simulink model "gm_uz_pmsm_model_9ph_working_vnl"  (R2021a)
settings: Solver=FixedStepAuto  StartTime=0.0  StopTime=0.04  RelTol=1e-3
PreLoadFcn:
  | uz_pmsm_model_9ph_init_parameter
undefined symbols (not defined in the file or in its folder): a, b, c, friction_coefficient, inertia, k_i_d, k_p_d, k_p_q, L_d, L_o1, L_o2, L_q, L_x1, L_x2, L_y1, L_y2, L_zero, polepair, psi_pm, R_1, static_friction_torque, ts
libraries: hdlmdlgenlib x182, hdlsllib x92, simulink x15, pid_lib x2
(part 3 of 5)

== system gm_uz_pmsm_model_9ph_working_vnl/Compare/Assert_out_theta_el ==
  cosim : Inport
  dut : Inport  Port=2
  AssertEq : Assertion  StopWhenAssertionFail=off
  Compare To Zero : simulink/Logic and Bit Operations/Compare To Zero  relop===  OutDataTypeStr=boolean
  Constant1 : Constant  Value=0  OutDataTypeStr=Inherit: Inherit via back propagation  SampleTime=-1
  Counter : simulink/Sources/Counter Free-Running  NumBits=32  tsamp=-1
  IgnoreCycles : Constant  Value=2  OutDataTypeStr=Inherit: Inherit via back propagation  SampleTime=-1
  Relational Operator : RelationalOperator  Operator=<  OutDataTypeStr=boolean  RndMeth=Nearest
  Relational Operator1 : RelationalOperator  Operator===  OutDataTypeStr=boolean  RndMeth=Nearest
  Switch : Switch  Criteria=u2 ~= 0
  Switch1 : Switch  Criteria=u2 ~= 0
  compare: out_theta_el : Scope  NumInputPorts=3
  wires:
  Compare To Zero/1 -> compare: out_theta_el/3
  Relational Operator1/1 -> Compare To Zero/1, AssertEq/1  "err"
  Switch1/1 -> compare: out_theta_el/1, Relational Operator1/1
  Switch/1 -> compare: out_theta_el/2, Relational Operator1/2
  Constant1/1 -> Switch/1, Switch1/1
  Relational Operator/1 -> Switch/2, Switch1/2
  cosim/1 -> Switch1/3  "cosim"
  dut/1 -> Switch/3  "dut ref"
  Counter/1 -> Relational Operator/1
  IgnoreCycles/1 -> Relational Operator/2

== system gm_uz_pmsm_model_9ph_working_vnl/Compare/Assert_outputs ==
  cosim : Inport
  dut : Inport  Port=2
  AssertEq : Assertion  StopWhenAssertionFail=off
  Compare To Zero : simulink/Logic and Bit Operations/Compare To Zero  relop===  OutDataTypeStr=boolean
  Constant1 : Constant  Value=0  OutDataTypeStr=Inherit: Inherit via back propagation  SampleTime=-1
  Counter : simulink/Sources/Counter Free-Running  NumBits=32  tsamp=-1
  IgnoreCycles : Constant  Value=2  OutDataTypeStr=Inherit: Inherit via back propagation  SampleTime=-1
  RelErrCheck : Subsystem
  Relational Operator : RelationalOperator  Operator=<  OutDataTypeStr=boolean  RndMeth=Nearest
  Switch : Switch  Criteria=u2 ~= 0
  Switch1 : Switch  Criteria=u2 ~= 0
  compare: outputs : Scope  NumInputPorts=3
  wires:
  IgnoreCycles/1 -> Relational Operator/2
  Counter/1 -> Relational Operator/1
  dut/1 -> Switch/3  "dut ref"
  cosim/1 -> Switch1/3  "cosim"
  Relational Operator/1 -> Switch1/2, Switch/2
  Constant1/1 -> Switch1/1, Switch/1
  Switch/1 -> compare: outputs/2, RelErrCheck/2(In2)
  Switch1/1 -> compare: outputs/1, RelErrCheck/1(In1)
  RelErrCheck/1(Out1) -> AssertEq/1, Compare To Zero/1  "err"
  Compare To Zero/1 -> compare: outputs/3

== system gm_uz_pmsm_model_9ph_working_vnl/Compare/CleanupScopes ==

== system gm_uz_pmsm_model_9ph_working_vnl/Compare/Enable ==

== system gm_uz_pmsm_model_9ph_working_vnl/FOC_controller/decoupling ==
  i_d : Inport
  i_q : Inport  Port=2
  omega_m : Inport  Port=3
  Constant1 : Constant  Value=psi_pm  SampleTime=-1
  Gain : Gain  Gain=L_q
  Gain1 : Gain  Gain=L_d
  Gain2 : Gain  Gain=polepair
  Product : Product
  Product1 : Product
  Sum6 : Sum  Inputs=|++
  u_d : Outport
  u_q : Outport  Port=2
  wires:
  Gain/1 -> Product/1
  Gain2/1 -> Product1/2, Product/2
  Product1/1 -> u_q/1
  i_d/1 -> Gain1/1
  Product/1 -> u_d/1
  Gain1/1 -> Sum6/1
  i_q/1 -> Gain/1
  Constant1/1 -> Sum6/2
  Sum6/1 -> Product1/1
  omega_m/1 -> Gain2/1

== system gm_uz_pmsm_model_9ph_working_vnl/uz_pmsm_model_9ph/Add ==
  In1 : Inport
  In2 : Inport  Port=2
  Add : Sum  Inputs=+-  OutDataTypeStr=single  SampleTime=2e-09
  Add_pd1 : Delay  DelayLength=6
  Out1 : Outport
  wires:
  Add_pd1/1 -> Out1/1
  Add/1 -> Add_pd1/1
  In2/1 -> Add/2
  In1/1 -> Add/1

== system gm_uz_pmsm_model_9ph_working_vnl/uz_pmsm_model_9ph/Add1 ==
  In1 : Inport
  In2 : Inport  Port=2
  Add1 : Sum  Inputs=+-  OutDataTypeStr=single  SampleTime=2e-09
  Add1_pd1 : Delay  DelayLength=6
  Out1 : Outport
  wires:
  Add1_pd1/1 -> Out1/1
  Add1/1 -> Add1_pd1/1
  In2/1 -> Add1/2
  In1/1 -> Add1/1

== system gm_uz_pmsm_model_9ph_working_vnl/uz_pmsm_model_9ph/Add2 ==
  In1 : Inport
  In2 : Inport  Port=2
  Add2 : Sum  Inputs=+-  OutDataTypeStr=single  SampleTime=2e-09
  Add2_pd1 : Delay  DelayLength=6
  Out1 : Outport
  wires:
  Add2_pd1/1 -> Out1/1
  Add2/1 -> Add2_pd1/1
  In2/1 -> Add2/2
  In1/1 -> Add2/1

== system gm_uz_pmsm_model_9ph_working_vnl/uz_pmsm_model_9ph/Add3 ==
  In1 : Inport
  In2 : Inport  Port=2
  Add3 : Sum  Inputs=+-  OutDataTypeStr=single  SampleTime=2e-09
  Add3_pd1 : Delay  DelayLength=6
  Out1 : Outport
  wires:
  Add3_pd1/1 -> Out1/1
  Add3/1 -> Add3_pd1/1
  In2/1 -> Add3/2
  In1/1 -> Add3/1

== system gm_uz_pmsm_model_9ph_working_vnl/uz_pmsm_model_9ph/Add4 ==
  In1 : Inport
  In2 : Inport  Port=2
  Add4 : Sum  Inputs=+-  OutDataTypeStr=single  SampleTime=2e-09
  Add4_pd1 : Delay  DelayLength=6
  Out1 : Outport
  wires:
  Add4_pd1/1 -> Out1/1
  Add4/1 -> Add4_pd1/1
  In2/1 -> Add4/2
  In1/1 -> Add4/1

== system gm_uz_pmsm_model_9ph_working_vnl/uz_pmsm_model_9ph/Add5 ==
  In1 : Inport
  In2 : Inport  Port=2
  Add5 : Sum  Inputs=+-  OutDataTypeStr=single  SampleTime=2e-09
  Add5_pd1 : Delay  DelayLength=6
  Out1 : Outport
  wires:
  Add5_pd1/1 -> Out1/1
  Add5/1 -> Add5_pd1/1
  In2/1 -> Add5/2
  In1/1 -> Add5/1

== system gm_uz_pmsm_model_9ph_working_vnl/uz_pmsm_model_9ph/Add6 ==
  In1 : Inport
  In2 : Inport  Port=2
  Add6 : Sum  Inputs=+-  OutDataTypeStr=single  SampleTime=2e-09
  Add6_pd1 : Delay  DelayLength=6
  Out1 : Outport
  wires:
  Add6_pd1/1 -> Out1/1
  Add6/1 -> Add6_pd1/1
  In2/1 -> Add6/2
  In1/1 -> Add6/1

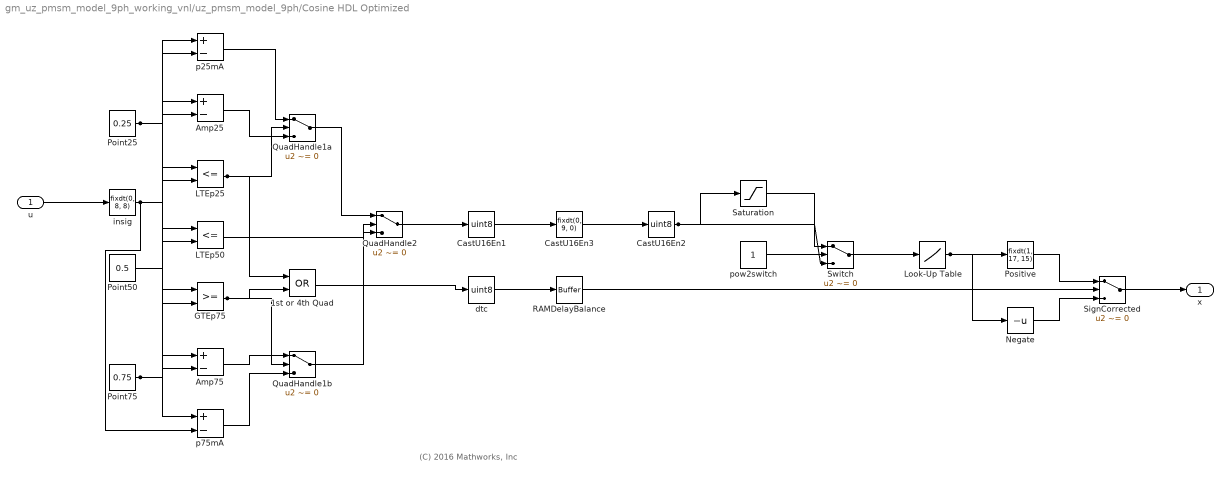
== system gm_uz_pmsm_model_9ph_working_vnl/uz_pmsm_model_9ph/Cosine HDL Optimized ==
  note: (C) 2016 Mathworks, Inc
  u : Inport  OutDataTypeStr=fixdt(1, 25, 12)  SampleTime=2e-09
  1st or 4th Quad : Logic  Operator=OR  AllPortsSameDT=off  OutDataTypeStr=boolean  SampleTime=2e-09
  Amp25 : Sum  Inputs=+-  AccumDataTypeStr=fixdt(1, 18, 17)  OutDataTypeStr=fixdt(1, 18, 17)  SampleTime=2e-09
  Amp75 : Sum  Inputs=+-  AccumDataTypeStr=fixdt(1, 18, 17)  OutDataTypeStr=fixdt(1, 18, 17)  SampleTime=2e-09
  CastU16En1 : DataTypeConversion  OutDataTypeStr=uint8  ConvertRealWorld=Stored Integer (SI)  SampleTime=2e-09
  CastU16En2 : DataTypeConversion  OutDataTypeStr=uint8  ConvertRealWorld=Stored Integer (SI)  SampleTime=2e-09  SaturateOnIntegerOverflow=on
  CastU16En3 : DataTypeConversion  OutDataTypeStr=fixdt(0, 9, 0)  SampleTime=2e-09
  GTEp75 : RelationalOperator  OutDataTypeStr=boolean  SampleTime=2e-09  RndMeth=Nearest
  LTEp25 : RelationalOperator  Operator=<=  OutDataTypeStr=boolean  SampleTime=2e-09  RndMeth=Nearest
  LTEp50 : RelationalOperator  Operator=<=  OutDataTypeStr=boolean  SampleTime=2e-09  RndMeth=Nearest
  Look-Up Table : Lookup_n-D  NumberOfTableDimensions=1  BreakpointsForDimension1="fi(\"numerictype\",numerictype(0,8,0),\"fimath\",fimath(\"RoundingMethod\", \"Floor\",\"OverflowAction\", \"Wrap\",\"ProductMode\",\"FullPrecision\",\"SumMode\",\"FullPrecision\"),\"Value\",\"[0 1 2 3 4 5 6 7 8 9 10 11 12 13 14 15 16 17 18 19 20 21 22 23 24 25 26 27 28 29 30 31 32 33 34 35 36 37 38 39 40 41 42 43 44 45 46 47 48 49 50 51 52 53 54 55 56 57 58 59 60 61 62 63]\")"  Table="reshape(fi(\"numerictype\",numerictype(1,17,15),\"fimath\",fimath(\"RoundingMethod\", \"Floor\",\"OverflowAction\", \"Wrap\",\"ProductMode\",\"FullPrecision\",\"SumMode\",\"FullPrecision\"),\"Value\",\"[0;0.0245361328125;0.049072265625;0.073577880859375;0.0980224609375;0.122406005859375;0.146728515625;0.17095947265625;0.195098876953125;0.2191162109375;0.24298095703125;0.2667236328125;0.290283203125;0.313690185546875;0.336883544921875;0.359893798828125;0.3826904296875;0.405242919921875;0.42755126953125;0.449615478515625;0.471405029296875;0.492889404296875;0.51409912109375;0.535003662109375;0.555572509765625;0.5758056640625;0.595703125;0.615234375;0.6343994140625;0.653167724609375;0.67156982421875;0.689544677734375;0.70709228515625;0.7242431640625;0.740936279296875;0.7572021484375;0.77301025390625;0.788360595703125;0.80322265625;0.817596435546875;0.83148193359375;0.8448486328125;0.85772705078125;0.870086669921875;0.881927490234375;0.893218994140625;0.90399169921875;0.914215087890625;0.92388916015625;0.9329833984375;0.941558837890625;0.94952392578125;0.956939697265625;0.963775634765625;0.97003173828125;0.9757080078125;0.98077392578125;0.98529052734375;0.989166259765625;0.99249267578125;0.99517822265625;0.997283935546875;0.998809814453125;0.99969482421875]\"), [1  64])"  InterpMethod=Flat  ExtrapMethod=Clip  DiagnosticForOutOfRangeInput=Error  SampleTime=2e-09  OutDataTypeStr=fixdt(1, 17, 15)  InputSameDT=on
  Negate : UnaryMinus  SampleTime=2e-09
  Point25 : Constant  Value=0.25  OutDataTypeStr=fixdt(0, 17, 17)  SampleTime=2e-09
  Point50 : Constant  Value=0.5  OutDataTypeStr=fixdt(0, 17, 17)  SampleTime=2e-09
  Point75 : Constant  Value=0.75  OutDataTypeStr=fixdt(0, 17, 17)  SampleTime=2e-09
  Positive : DataTypeConversion  OutDataTypeStr=fixdt(1, 17, 15)  SampleTime=2e-09
  QuadHandle1a : Switch  Criteria=u2 ~= 0  Threshold=double(0)  OutDataTypeStr=fixdt(1, 18, 17)  SampleTime=2e-09
  QuadHandle1b : Switch  Criteria=u2 ~= 0  Threshold=double(0)  OutDataTypeStr=fixdt(1, 18, 17)  SampleTime=2e-09
  QuadHandle2 : Switch  Criteria=u2 ~= 0  Threshold=double(0)  OutDataTypeStr=fixdt(0, 8, 8)  SampleTime=2e-09  SaturateOnIntegerOverflow=on
  RAMDelayBalance : hdlmdlgenlib/Buffer
      settings: SourceProductBaseCode=SL
  Saturation : Saturate  UpperLimit="fi(0,0,8,0,\"hex\",\"3f\")"  LowerLimit="fi(0,0,8,0,\"hex\",\"00\")"  SampleTime=2e-09  OutDataTypeStr=uint8
  SignCorrected : Switch  Criteria=u2 ~= 0  Threshold=double(0)  OutDataTypeStr=fixdt(1, 17, 15)  SampleTime=2e-09
  Switch : Switch  Criteria=u2 ~= 0  Threshold=double(0)  OutDataTypeStr=uint8  SampleTime=2e-09
  dtc : DataTypeConversion  OutDataTypeStr=uint8  SampleTime=2e-09
  insig : DataTypeConversion  OutDataTypeStr=fixdt(0, 8, 8)  SampleTime=2e-09
  p25mA : Sum  Inputs=+-  AccumDataTypeStr=fixdt(1, 18, 17)  OutDataTypeStr=fixdt(1, 18, 17)  SampleTime=2e-09
  p75mA : Sum  Inputs=+-  AccumDataTypeStr=fixdt(1, 18, 17)  OutDataTypeStr=fixdt(1, 18, 17)  SampleTime=2e-09
  pow2switch : Constant  OutDataTypeStr=boolean  SampleTime=2e-09
  x : Outport  SampleTime=2e-09
  wires:
  u/1 -> insig/1
  1st or 4th Quad/1 -> dtc/1
  pow2switch/1 -> Switch/2
  p75mA/1 -> QuadHandle1b/3
  p25mA/1 -> QuadHandle1a/1
  insig/1 -> Amp25/1, Amp75/1, GTEp75/1, LTEp25/1, LTEp50/1, p25mA/2, p75mA/2
  Switch/1 -> Look-Up Table/1
  SignCorrected/1 -> x/1
  Saturation/1 -> Switch/1
  RAMDelayBalance/1 -> SignCorrected/2
  QuadHandle2/1 -> CastU16En1/1
  QuadHandle1b/1 -> QuadHandle2/3
  QuadHandle1a/1 -> QuadHandle2/1
  Positive/1 -> SignCorrected/1
  Point75/1 -> Amp75/2, GTEp75/2, p75mA/1
  Point50/1 -> LTEp50/2
  Point25/1 -> Amp25/2, LTEp25/2, p25mA/1
  Negate/1 -> SignCorrected/3
  Look-Up Table/1 -> Negate/1, Positive/1
  LTEp50/1 -> QuadHandle2/2
  LTEp25/1 -> 1st or 4th Quad/1, QuadHandle1a/2
  GTEp75/1 -> 1st or 4th Quad/2, QuadHandle1b/2
  CastU16En3/1 -> CastU16En2/1
  CastU16En2/1 -> Saturation/1, Switch/3
  CastU16En1/1 -> CastU16En3/1
  Amp75/1 -> QuadHandle1b/1
  Amp25/1 -> QuadHandle1a/3
  dtc/1 -> RAMDelayBalance/1

== system gm_uz_pmsm_model_9ph_working_vnl/uz_pmsm_model_9ph/Data Type Conversion1 ==
  In1 : Inport
  Data Type Conversion1 : DataTypeConversion  OutDataTypeStr=fixdt(1, 25, 12)  RndMeth=Nearest  SampleTime=2e-09
  Data Type Conversion1_pd1 : Delay  DelayLength=6
  Out1 : Outport
  wires:
  Data Type Conversion1_pd1/1 -> Out1/1
  Data Type Conversion1/1 -> Data Type Conversion1_pd1/1
  In1/1 -> Data Type Conversion1/1

== system gm_uz_pmsm_model_9ph_working_vnl/uz_pmsm_model_9ph/Data Type Conversion11 ==
  In1 : Inport
  Data Type Conversion11 : DataTypeConversion  OutDataTypeStr=double  RndMeth=Nearest  SampleTime=2e-09
  Data Type Conversion11_pd1 : Delay  DelayLength=3
  Out1 : Outport
  wires:
  Data Type Conversion11_pd1/1 -> Out1/1
  Data Type Conversion11/1 -> Data Type Conversion11_pd1/1
  In1/1 -> Data Type Conversion11/1

== system gm_uz_pmsm_model_9ph_working_vnl/uz_pmsm_model_9ph/Data Type Conversion13 ==
  In1 : Inport
  Data Type Conversion13 : DataTypeConversion  OutDataTypeStr=single  RndMeth=Nearest  SampleTime=2e-09
  Data Type Conversion13_pd1 : Delay  DelayLength=3
  Out1 : Outport
  wires:
  Data Type Conversion13_pd1/1 -> Out1/1
  Data Type Conversion13/1 -> Data Type Conversion13_pd1/1
  In1/1 -> Data Type Conversion13/1

== system gm_uz_pmsm_model_9ph_working_vnl/uz_pmsm_model_9ph/Data Type Conversion14 ==
  In1 : Inport
  Data Type Conversion14 : DataTypeConversion  OutDataTypeStr=single  RndMeth=Nearest  SampleTime=2e-09
  Data Type Conversion14_pd1 : Delay  DelayLength=3
  Out1 : Outport
  wires:
  Data Type Conversion14_pd1/1 -> Out1/1
  Data Type Conversion14/1 -> Data Type Conversion14_pd1/1
  In1/1 -> Data Type Conversion14/1

== system gm_uz_pmsm_model_9ph_working_vnl/uz_pmsm_model_9ph/Data Type Conversion15 ==
  In1 : Inport
  Data Type Conversion15 : DataTypeConversion  OutDataTypeStr=single  RndMeth=Nearest  SampleTime=2e-09
  Data Type Conversion15_pd1 : Delay  DelayLength=3
  Out1 : Outport
  wires:
  Data Type Conversion15_pd1/1 -> Out1/1
  Data Type Conversion15/1 -> Data Type Conversion15_pd1/1
  In1/1 -> Data Type Conversion15/1

== system gm_uz_pmsm_model_9ph_working_vnl/uz_pmsm_model_9ph/Data Type Conversion16 ==
  In1 : Inport
  Data Type Conversion16 : DataTypeConversion  OutDataTypeStr=single  RndMeth=Nearest  SampleTime=2e-09
  Data Type Conversion16_pd1 : Delay  DelayLength=3
  Out1 : Outport
  wires:
  Data Type Conversion16_pd1/1 -> Out1/1
  Data Type Conversion16/1 -> Data Type Conversion16_pd1/1
  In1/1 -> Data Type Conversion16/1

== system gm_uz_pmsm_model_9ph_working_vnl/uz_pmsm_model_9ph/Data Type Conversion17 ==
  In1 : Inport
  Data Type Conversion17 : DataTypeConversion  OutDataTypeStr=single  RndMeth=Nearest  SampleTime=2e-09
  Data Type Conversion17_pd1 : Delay  DelayLength=3
  Out1 : Outport
  wires:
  Data Type Conversion17_pd1/1 -> Out1/1
  Data Type Conversion17/1 -> Data Type Conversion17_pd1/1
  In1/1 -> Data Type Conversion17/1

== system gm_uz_pmsm_model_9ph_working_vnl/uz_pmsm_model_9ph/Data Type Conversion18 ==
  In1 : Inport
  Data Type Conversion18 : DataTypeConversion  OutDataTypeStr=single  RndMeth=Nearest  SampleTime=2e-09
  Data Type Conversion18_pd1 : Delay  DelayLength=3
  Out1 : Outport
  wires:
  Data Type Conversion18_pd1/1 -> Out1/1
  Data Type Conversion18/1 -> Data Type Conversion18_pd1/1
  In1/1 -> Data Type Conversion18/1

== system gm_uz_pmsm_model_9ph_working_vnl/uz_pmsm_model_9ph/Data Type Conversion19 ==
  In1 : Inport
  Data Type Conversion19 : DataTypeConversion  OutDataTypeStr=single  RndMeth=Nearest  SampleTime=2e-09
  Data Type Conversion19_pd1 : Delay  DelayLength=3
  Out1 : Outport
  wires:
  Data Type Conversion19_pd1/1 -> Out1/1
  Data Type Conversion19/1 -> Data Type Conversion19_pd1/1
  In1/1 -> Data Type Conversion19/1

== system gm_uz_pmsm_model_9ph_working_vnl/uz_pmsm_model_9ph/Data Type Conversion20 ==
  In1 : Inport
  Data Type Conversion20 : DataTypeConversion  OutDataTypeStr=single  RndMeth=Nearest  SampleTime=2e-09
  Data Type Conversion20_pd1 : Delay  DelayLength=3
  Out1 : Outport
  wires:
  Data Type Conversion20_pd1/1 -> Out1/1
  Data Type Conversion20/1 -> Data Type Conversion20_pd1/1
  In1/1 -> Data Type Conversion20/1

== system gm_uz_pmsm_model_9ph_working_vnl/uz_pmsm_model_9ph/Data Type Conversion21 ==
  In1 : Inport
  Data Type Conversion21 : DataTypeConversion  OutDataTypeStr=double  RndMeth=Nearest  SampleTime=2e-09
  Data Type Conversion21_pd1 : Delay  DelayLength=3
  Out1 : Outport
  wires:
  Data Type Conversion21_pd1/1 -> Out1/1
  Data Type Conversion21/1 -> Data Type Conversion21_pd1/1
  In1/1 -> Data Type Conversion21/1

== system gm_uz_pmsm_model_9ph_working_vnl/uz_pmsm_model_9ph/Data Type Conversion22 ==
  In1 : Inport
  Data Type Conversion22 : DataTypeConversion  OutDataTypeStr=single  RndMeth=Nearest  SampleTime=2e-09
  Data Type Conversion22_pd1 : Delay  DelayLength=6
  Out1 : Outport
  wires:
  Data Type Conversion22_pd1/1 -> Out1/1
  Data Type Conversion22/1 -> Data Type Conversion22_pd1/1
  In1/1 -> Data Type Conversion22/1

== system gm_uz_pmsm_model_9ph_working_vnl/uz_pmsm_model_9ph/Data Type Conversion221 ==
  In1 : Inport
  Data Type Conversion221 : DataTypeConversion  OutDataTypeStr=double  RndMeth=Nearest  SampleTime=2e-09
  Data Type Conversion221_pd1 : Delay  DelayLength=3
  Out1 : Outport
  wires:
  Data Type Conversion221_pd1/1 -> Out1/1
  Data Type Conversion221/1 -> Data Type Conversion221_pd1/1
  In1/1 -> Data Type Conversion221/1

== system gm_uz_pmsm_model_9ph_working_vnl/uz_pmsm_model_9ph/Data Type Conversion23 ==
  In1 : Inport
  Data Type Conversion23 : DataTypeConversion  OutDataTypeStr=single  RndMeth=Nearest  SampleTime=2e-09
  Data Type Conversion23_pd1 : Delay  DelayLength=3
  Out1 : Outport
  wires:
  Data Type Conversion23_pd1/1 -> Out1/1
  Data Type Conversion23/1 -> Data Type Conversion23_pd1/1
  In1/1 -> Data Type Conversion23/1

== system gm_uz_pmsm_model_9ph_working_vnl/uz_pmsm_model_9ph/Data Type Conversion24 ==
  In1 : Inport
  Data Type Conversion24 : DataTypeConversion  OutDataTypeStr=double  RndMeth=Nearest  SampleTime=2e-09
  Data Type Conversion24_pd1 : Delay  DelayLength=3
  Out1 : Outport
  wires:
  Data Type Conversion24_pd1/1 -> Out1/1
  Data Type Conversion24/1 -> Data Type Conversion24_pd1/1
  In1/1 -> Data Type Conversion24/1

== system gm_uz_pmsm_model_9ph_working_vnl/uz_pmsm_model_9ph/Data Type Conversion25 ==
  In1 : Inport
  Data Type Conversion25 : DataTypeConversion  OutDataTypeStr=double  RndMeth=Nearest  SampleTime=2e-09
  Data Type Conversion25_pd1 : Delay  DelayLength=3
  Out1 : Outport
  wires:
  Data Type Conversion25_pd1/1 -> Out1/1
  Data Type Conversion25/1 -> Data Type Conversion25_pd1/1
  In1/1 -> Data Type Conversion25/1

== system gm_uz_pmsm_model_9ph_working_vnl/uz_pmsm_model_9ph/Data Type Conversion26 ==
  In1 : Inport
  Data Type Conversion26 : DataTypeConversion  OutDataTypeStr=double  RndMeth=Nearest  SampleTime=2e-09
  Data Type Conversion26_pd1 : Delay  DelayLength=3
  Out1 : Outport
  wires:
  Data Type Conversion26_pd1/1 -> Out1/1
  Data Type Conversion26/1 -> Data Type Conversion26_pd1/1
  In1/1 -> Data Type Conversion26/1

== system gm_uz_pmsm_model_9ph_working_vnl/uz_pmsm_model_9ph/Data Type Conversion27 ==
  In1 : Inport
  Data Type Conversion27 : DataTypeConversion  OutDataTypeStr=double  RndMeth=Nearest  SampleTime=2e-09
  Data Type Conversion27_pd1 : Delay  DelayLength=3
  Out1 : Outport
  wires:
  Data Type Conversion27_pd1/1 -> Out1/1
  Data Type Conversion27/1 -> Data Type Conversion27_pd1/1
  In1/1 -> Data Type Conversion27/1

== system gm_uz_pmsm_model_9ph_working_vnl/uz_pmsm_model_9ph/Data Type Conversion28 ==
  In1 : Inport
  Data Type Conversion28 : DataTypeConversion  OutDataTypeStr=double  RndMeth=Nearest  SampleTime=2e-09
  Data Type Conversion28_pd1 : Delay  DelayLength=3
  Out1 : Outport
  wires:
  Data Type Conversion28_pd1/1 -> Out1/1
  Data Type Conversion28/1 -> Data Type Conversion28_pd1/1
  In1/1 -> Data Type Conversion28/1

== system gm_uz_pmsm_model_9ph_working_vnl/uz_pmsm_model_9ph/Data Type Conversion29 ==
  In1 : Inport
  Data Type Conversion29 : DataTypeConversion  OutDataTypeStr=double  RndMeth=Nearest  SampleTime=2e-09
  Data Type Conversion29_pd1 : Delay  DelayLength=3
  Out1 : Outport
  wires:
  Data Type Conversion29_pd1/1 -> Out1/1
  Data Type Conversion29/1 -> Data Type Conversion29_pd1/1
  In1/1 -> Data Type Conversion29/1

== system gm_uz_pmsm_model_9ph_working_vnl/uz_pmsm_model_9ph/Data Type Conversion30 ==
  In1 : Inport
  Data Type Conversion30 : DataTypeConversion  OutDataTypeStr=double  RndMeth=Nearest  SampleTime=2e-09
  Data Type Conversion30_pd1 : Delay  DelayLength=3
  Out1 : Outport
  wires:
  Data Type Conversion30_pd1/1 -> Out1/1
  Data Type Conversion30/1 -> Data Type Conversion30_pd1/1
  In1/1 -> Data Type Conversion30/1

== system gm_uz_pmsm_model_9ph_working_vnl/uz_pmsm_model_9ph/Data Type Conversion32 ==
  In1 : Inport
  Data Type Conversion32 : DataTypeConversion  OutDataTypeStr=single  RndMeth=Nearest  SampleTime=2e-09
  Data Type Conversion32_pd1 : Delay  DelayLength=6
  Out1 : Outport
  wires:
  Data Type Conversion32_pd1/1 -> Out1/1
  Data Type Conversion32/1 -> Data Type Conversion32_pd1/1
  In1/1 -> Data Type Conversion32/1

== system gm_uz_pmsm_model_9ph_working_vnl/uz_pmsm_model_9ph/Data Type Conversion8 ==
  In1 : Inport
  Data Type Conversion8 : DataTypeConversion  OutDataTypeStr=single  RndMeth=Nearest  SampleTime=2e-09
  Data Type Conversion8_pd1 : Delay  DelayLength=3
  Out1 : Outport
  wires:
  Data Type Conversion8_pd1/1 -> Out1/1
  Data Type Conversion8/1 -> Data Type Conversion8_pd1/1
  In1/1 -> Data Type Conversion8/1

== system gm_uz_pmsm_model_9ph_working_vnl/uz_pmsm_model_9ph/Divide ==
  In1 : Inport
  In2 : Inport  Port=2
  Divide : Product  Inputs=**  OutDataTypeStr=single  SampleTime=2e-09
  Divide_pd1 : Delay  DelayLength=6
  Out1 : Outport
  wires:
  Divide_pd1/1 -> Out1/1
  Divide/1 -> Divide_pd1/1
  In2/1 -> Divide/2
  In1/1 -> Divide/1

== system gm_uz_pmsm_model_9ph_working_vnl/uz_pmsm_model_9ph/Divide1 ==
  In1 : Inport
  In2 : Inport  Port=2
  Divide1 : Product  Inputs=**  OutDataTypeStr=single  SampleTime=2e-09
  Divide1_pd1 : Delay  DelayLength=6
  Out1 : Outport
  wires:
  Divide1_pd1/1 -> Out1/1
  Divide1/1 -> Divide1_pd1/1
  In2/1 -> Divide1/2
  In1/1 -> Divide1/1

== system gm_uz_pmsm_model_9ph_working_vnl/uz_pmsm_model_9ph/Divide10 ==
  In1 : Inport
  In2 : Inport  Port=2
  Divide10 : Product  Inputs=**  OutDataTypeStr=single  SampleTime=2e-09
  Divide10_pd1 : Delay  DelayLength=6
  Out1 : Outport
  wires:
  Divide10_pd1/1 -> Out1/1
  Divide10/1 -> Divide10_pd1/1
  In2/1 -> Divide10/2
  In1/1 -> Divide10/1

== system gm_uz_pmsm_model_9ph_working_vnl/uz_pmsm_model_9ph/Divide11 ==
  In1 : Inport
  In2 : Inport  Port=2
  Divide11 : Product  Inputs=**  OutDataTypeStr=single  SampleTime=2e-09
  Divide11_pd1 : Delay  DelayLength=6
  Out1 : Outport
  wires:
  Divide11_pd1/1 -> Out1/1
  Divide11/1 -> Divide11_pd1/1
  In2/1 -> Divide11/2
  In1/1 -> Divide11/1

== system gm_uz_pmsm_model_9ph_working_vnl/uz_pmsm_model_9ph/Divide12 ==
  In1 : Inport
  In2 : Inport  Port=2
  Divide12 : Product  Inputs=**  OutDataTypeStr=single  SampleTime=2e-09
  Divide12_pd1 : Delay  DelayLength=6
  Out1 : Outport
  wires:
  Divide12_pd1/1 -> Out1/1
  Divide12/1 -> Divide12_pd1/1
  In2/1 -> Divide12/2
  In1/1 -> Divide12/1

== system gm_uz_pmsm_model_9ph_working_vnl/uz_pmsm_model_9ph/Divide13 ==
  In1 : Inport
  In2 : Inport  Port=2
  Divide13 : Product  Inputs=**  OutDataTypeStr=single  SampleTime=2e-09
  Divide13_pd1 : Delay  DelayLength=6
  Out1 : Outport
  wires:
  Divide13_pd1/1 -> Out1/1
  Divide13/1 -> Divide13_pd1/1
  In2/1 -> Divide13/2
  In1/1 -> Divide13/1

== system gm_uz_pmsm_model_9ph_working_vnl/uz_pmsm_model_9ph/Divide2 ==
  In1 : Inport
  In2 : Inport  Port=2
  Divide2 : Product  Inputs=**  OutDataTypeStr=single  SampleTime=2e-09
  Divide2_pd1 : Delay  DelayLength=6
  Out1 : Outport
  wires:
  Divide2_pd1/1 -> Out1/1
  Divide2/1 -> Divide2_pd1/1
  In2/1 -> Divide2/2
  In1/1 -> Divide2/1

== system gm_uz_pmsm_model_9ph_working_vnl/uz_pmsm_model_9ph/Divide3 ==
  In1 : Inport
  In2 : Inport  Port=2
  Divide3 : Product  Inputs=**  OutDataTypeStr=single  SampleTime=2e-09
  Divide3_pd1 : Delay  DelayLength=6
  Out1 : Outport
  wires:
  Divide3_pd1/1 -> Out1/1
  Divide3/1 -> Divide3_pd1/1
  In2/1 -> Divide3/2
  In1/1 -> Divide3/1

== system gm_uz_pmsm_model_9ph_working_vnl/uz_pmsm_model_9ph/Divide4 ==
  In1 : Inport
  In2 : Inport  Port=2
  Divide4 : Product  Inputs=**  OutDataTypeStr=single  SampleTime=2e-09
  Divide4_pd1 : Delay  DelayLength=6
  Out1 : Outport
  wires:
  Divide4_pd1/1 -> Out1/1
  Divide4/1 -> Divide4_pd1/1
  In2/1 -> Divide4/2
  In1/1 -> Divide4/1

== system gm_uz_pmsm_model_9ph_working_vnl/uz_pmsm_model_9ph/Divide5 ==
  In1 : Inport
  In2 : Inport  Port=2
  Divide5 : Product  Inputs=**  OutDataTypeStr=single  SampleTime=2e-09
  Divide5_pd1 : Delay  DelayLength=6
  Out1 : Outport
  wires:
  Divide5_pd1/1 -> Out1/1
  Divide5/1 -> Divide5_pd1/1
  In2/1 -> Divide5/2
  In1/1 -> Divide5/1

== system gm_uz_pmsm_model_9ph_working_vnl/uz_pmsm_model_9ph/Divide6 ==
  In1 : Inport
  In2 : Inport  Port=2
  Divide6 : Product  Inputs=**  OutDataTypeStr=single  SampleTime=2e-09
  Divide6_pd1 : Delay  DelayLength=6
  Out1 : Outport
  wires:
  Divide6_pd1/1 -> Out1/1
  Divide6/1 -> Divide6_pd1/1
  In2/1 -> Divide6/2
  In1/1 -> Divide6/1

== system gm_uz_pmsm_model_9ph_working_vnl/uz_pmsm_model_9ph/Divide7 ==
  In1 : Inport
  In2 : Inport  Port=2
  Divide7 : Product  Inputs=**  OutDataTypeStr=single  SampleTime=2e-09
  Divide7_pd1 : Delay  DelayLength=6
  Out1 : Outport
  wires:
  Divide7_pd1/1 -> Out1/1
  Divide7/1 -> Divide7_pd1/1
  In2/1 -> Divide7/2
  In1/1 -> Divide7/1

== system gm_uz_pmsm_model_9ph_working_vnl/uz_pmsm_model_9ph/Divide8 ==
  In1 : Inport
  In2 : Inport  Port=2
  Divide8 : Product  Inputs=**  OutDataTypeStr=single  SampleTime=2e-09
  Divide8_pd1 : Delay  DelayLength=6
  Out1 : Outport
  wires:
  Divide8_pd1/1 -> Out1/1
  Divide8/1 -> Divide8_pd1/1
  In2/1 -> Divide8/2
  In1/1 -> Divide8/1

== system gm_uz_pmsm_model_9ph_working_vnl/uz_pmsm_model_9ph/Divide9 ==
  In1 : Inport
  In2 : Inport  Port=2
  Divide9 : Product  Inputs=**  OutDataTypeStr=single  SampleTime=2e-09
  Divide9_pd1 : Delay  DelayLength=6
  Out1 : Outport
  wires:
  Divide9_pd1/1 -> Out1/1
  Divide9/1 -> Divide9_pd1/1
  In2/1 -> Divide9/2
  In1/1 -> Divide9/1

== system gm_uz_pmsm_model_9ph_working_vnl/uz_pmsm_model_9ph/Factor ==
  In1 : Inport
  In2 : Inport  Port=2
  Factor : Product  Inputs=**  OutDataTypeStr=single  SampleTime=2e-09
  Factor_pd1 : Delay  DelayLength=6
  Out1 : Outport
  wires:
  Factor_pd1/1 -> Out1/1
  Factor/1 -> Factor_pd1/1
  In2/1 -> Factor/2
  In1/1 -> Factor/1

== system gm_uz_pmsm_model_9ph_working_vnl/uz_pmsm_model_9ph/Gain ==
  In1 : Inport
  In2 : Inport  Port=2
  Gain : Product  Inputs=**  OutDataTypeStr=double  SampleTime=2e-09
  Gain_pd1 : Delay  DelayLength=6
  Out1 : Outport
  wires:
  Gain_pd1/1 -> Out1/1
  Gain/1 -> Gain_pd1/1
  In2/1 -> Gain/2
  In1/1 -> Gain/1

== system gm_uz_pmsm_model_9ph_working_vnl/uz_pmsm_model_9ph/Gain1 ==
  In1 : Inport
  In2 : Inport  Port=2
  Gain1 : Product  Inputs=**  OutDataTypeStr=double  SampleTime=2e-09
  Gain1_pd1 : Delay  DelayLength=6
  Out1 : Outport
  wires:
  Gain1_pd1/1 -> Out1/1
  Gain1/1 -> Gain1_pd1/1
  In2/1 -> Gain1/2
  In1/1 -> Gain1/1

== system gm_uz_pmsm_model_9ph_working_vnl/uz_pmsm_model_9ph/Gain2 ==
  In1 : Inport
  In2 : Inport  Port=2
  Gain2 : Product  Inputs=**  OutDataTypeStr=double  SampleTime=2e-09
  Gain2_pd1 : Delay  DelayLength=6
  Out1 : Outport
  wires:
  Gain2_pd1/1 -> Out1/1
  Gain2/1 -> Gain2_pd1/1
  In2/1 -> Gain2/2
  In1/1 -> Gain2/1

== system gm_uz_pmsm_model_9ph_working_vnl/uz_pmsm_model_9ph/Gain3 ==
  In1 : Inport
  In2 : Inport  Port=2
  Gain3 : Product  Inputs=**  OutDataTypeStr=double  SampleTime=2e-09
  Gain3_pd1 : Delay  DelayLength=6
  Out1 : Outport
  wires:
  Gain3_pd1/1 -> Out1/1
  Gain3/1 -> Gain3_pd1/1
  In2/1 -> Gain3/2
  In1/1 -> Gain3/1

== system gm_uz_pmsm_model_9ph_working_vnl/uz_pmsm_model_9ph/Gain4 ==
  In1 : Inport
  In2 : Inport  Port=2
  Gain4 : Product  Inputs=**  OutDataTypeStr=double  SampleTime=2e-09
  Gain4_pd1 : Delay  DelayLength=6
  Out1 : Outport
  wires:
  Gain4_pd1/1 -> Out1/1
  Gain4/1 -> Gain4_pd1/1
  In2/1 -> Gain4/2
  In1/1 -> Gain4/1

== system gm_uz_pmsm_model_9ph_working_vnl/uz_pmsm_model_9ph/Gain5 ==
  In1 : Inport
  In2 : Inport  Port=2
  Gain5 : Product  Inputs=**  OutDataTypeStr=double  SampleTime=2e-09
  Gain5_pd1 : Delay  DelayLength=6
  Out1 : Outport
  wires:
  Gain5_pd1/1 -> Out1/1
  Gain5/1 -> Gain5_pd1/1
  In2/1 -> Gain5/2
  In1/1 -> Gain5/1

== system gm_uz_pmsm_model_9ph_working_vnl/uz_pmsm_model_9ph/Gain6 ==
  In1 : Inport
  In2 : Inport  Port=2
  Gain6 : Product  Inputs=**  OutDataTypeStr=double  SampleTime=2e-09
  Gain6_pd1 : Delay  DelayLength=6
  Out1 : Outport
  wires:
  Gain6_pd1/1 -> Out1/1
  Gain6/1 -> Gain6_pd1/1
  In2/1 -> Gain6/2
  In1/1 -> Gain6/1

== system gm_uz_pmsm_model_9ph_working_vnl/uz_pmsm_model_9ph/Gain7 ==
  In1 : Inport
  In2 : Inport  Port=2
  Gain7 : Product  Inputs=**  OutDataTypeStr=double  SampleTime=2e-09
  Gain7_pd1 : Delay  DelayLength=6
  Out1 : Outport
  wires:
  Gain7_pd1/1 -> Out1/1
  Gain7/1 -> Gain7_pd1/1
  In2/1 -> Gain7/2
  In1/1 -> Gain7/1

== system gm_uz_pmsm_model_9ph_working_vnl/uz_pmsm_model_9ph/Gain8 ==
  In1 : Inport
  In2 : Inport  Port=2
  Gain8 : Product  Inputs=**  OutDataTypeStr=double  SampleTime=2e-09
  Gain8_pd1 : Delay  DelayLength=6
  Out1 : Outport
  wires:
  Gain8_pd1/1 -> Out1/1
  Gain8/1 -> Gain8_pd1/1
  In2/1 -> Gain8/2
  In1/1 -> Gain8/1

== system gm_uz_pmsm_model_9ph_working_vnl/uz_pmsm_model_9ph/Gain9 ==
  In1 : Inport
  In2 : Inport  Port=2
  Gain9 : Product  Inputs=**  OutDataTypeStr=double  SampleTime=2e-09
  Gain9_pd1 : Delay  DelayLength=6
  Out1 : Outport
  wires:
  Gain9_pd1/1 -> Out1/1
  Gain9/1 -> Gain9_pd1/1
  In2/1 -> Gain9/2
  In1/1 -> Gain9/1

== system gm_uz_pmsm_model_9ph_working_vnl/uz_pmsm_model_9ph/Product ==
  In1 : Inport
  In2 : Inport  Port=2
  Product : Product  Inputs=**  OutDataTypeStr=single  SampleTime=2e-09
  Product_pd1 : Delay  DelayLength=6
  Out1 : Outport
  wires:
  Product_pd1/1 -> Out1/1
  Product/1 -> Product_pd1/1
  In2/1 -> Product/2
  In1/1 -> Product/1

== system gm_uz_pmsm_model_9ph_working_vnl/uz_pmsm_model_9ph/Product1 ==
  In1 : Inport
  In2 : Inport  Port=2
  Product1 : Product  Inputs=**  OutDataTypeStr=single  SampleTime=2e-09
  Product1_pd1 : Delay  DelayLength=6
  Out1 : Outport
  wires:
  Product1_pd1/1 -> Out1/1
  Product1/1 -> Product1_pd1/1
  In2/1 -> Product1/2
  In1/1 -> Product1/1

== system gm_uz_pmsm_model_9ph_working_vnl/uz_pmsm_model_9ph/Product10 ==
  In1 : Inport
  In2 : Inport  Port=2
  Product10 : Product  Inputs=**  OutDataTypeStr=single  SampleTime=2e-09
  Product10_pd1 : Delay  DelayLength=6
  Out1 : Outport
  wires:
  Product10_pd1/1 -> Out1/1
  Product10/1 -> Product10_pd1/1
  In2/1 -> Product10/2
  In1/1 -> Product10/1

== system gm_uz_pmsm_model_9ph_working_vnl/uz_pmsm_model_9ph/Product11 ==
  In1 : Inport
  In2 : Inport  Port=2
  Product11 : Product  Inputs=**  OutDataTypeStr=single  SampleTime=2e-09
  Product11_pd1 : Delay  DelayLength=6
  Out1 : Outport
  wires:
  Product11_pd1/1 -> Out1/1
  Product11/1 -> Product11_pd1/1
  In2/1 -> Product11/2
  In1/1 -> Product11/1

== system gm_uz_pmsm_model_9ph_working_vnl/uz_pmsm_model_9ph/Product2 ==
  In1 : Inport
  In2 : Inport  Port=2
  Product2 : Product  Inputs=**  OutDataTypeStr=single  SampleTime=2e-09
  Product2_pd1 : Delay  DelayLength=6
  Out1 : Outport
  wires:
  Product2_pd1/1 -> Out1/1
  Product2/1 -> Product2_pd1/1
  In2/1 -> Product2/2
  In1/1 -> Product2/1

== system gm_uz_pmsm_model_9ph_working_vnl/uz_pmsm_model_9ph/Product3 ==
  In1 : Inport
  In2 : Inport  Port=2
  Product3 : Product  Inputs=**  OutDataTypeStr=single  SampleTime=2e-09
  Product3_pd1 : Delay  DelayLength=6
  Out1 : Outport
  wires:
  Product3_pd1/1 -> Out1/1
  Product3/1 -> Product3_pd1/1
  In2/1 -> Product3/2
  In1/1 -> Product3/1

== system gm_uz_pmsm_model_9ph_working_vnl/uz_pmsm_model_9ph/Product5 ==
  In1 : Inport
  In2 : Inport  Port=2
  Product5 : Product  Inputs=**  OutDataTypeStr=single  SampleTime=2e-09
  Product5_pd1 : Delay  DelayLength=6
  Out1 : Outport
  wires:
  Product5_pd1/1 -> Out1/1
  Product5/1 -> Product5_pd1/1
  In2/1 -> Product5/2
  In1/1 -> Product5/1

== system gm_uz_pmsm_model_9ph_working_vnl/uz_pmsm_model_9ph/Product6 ==
  In1 : Inport
  In2 : Inport  Port=2
  Product6 : Product  Inputs=**  OutDataTypeStr=single  SampleTime=2e-09
  Product6_pd1 : Delay  DelayLength=6
  Out1 : Outport
  wires:
  Product6_pd1/1 -> Out1/1
  Product6/1 -> Product6_pd1/1
  In2/1 -> Product6/2
  In1/1 -> Product6/1

== system gm_uz_pmsm_model_9ph_working_vnl/uz_pmsm_model_9ph/Product7 ==
  In1 : Inport
  In2 : Inport  Port=2
  Product7 : Product  Inputs=**  OutDataTypeStr=single  SampleTime=2e-09
  Product7_pd1 : Delay  DelayLength=6
  Out1 : Outport
  wires:
  Product7_pd1/1 -> Out1/1
  Product7/1 -> Product7_pd1/1
  In2/1 -> Product7/2
  In1/1 -> Product7/1

== system gm_uz_pmsm_model_9ph_working_vnl/uz_pmsm_model_9ph/Product8 ==
  In1 : Inport
  In2 : Inport  Port=2
  Product8 : Product  Inputs=**  OutDataTypeStr=single  SampleTime=2e-09
  Product8_pd1 : Delay  DelayLength=6
  Out1 : Outport
  wires:
  Product8_pd1/1 -> Out1/1
  Product8/1 -> Product8_pd1/1
  In2/1 -> Product8/2
  In1/1 -> Product8/1

== system gm_uz_pmsm_model_9ph_working_vnl/uz_pmsm_model_9ph/Product9 ==
  In1 : Inport
  In2 : Inport  Port=2
  Product9 : Product  Inputs=**  OutDataTypeStr=single  SampleTime=2e-09
  Product9_pd1 : Delay  DelayLength=6
  Out1 : Outport
  wires:
  Product9_pd1/1 -> Out1/1
  Product9/1 -> Product9_pd1/1
  In2/1 -> Product9/2
  In1/1 -> Product9/1

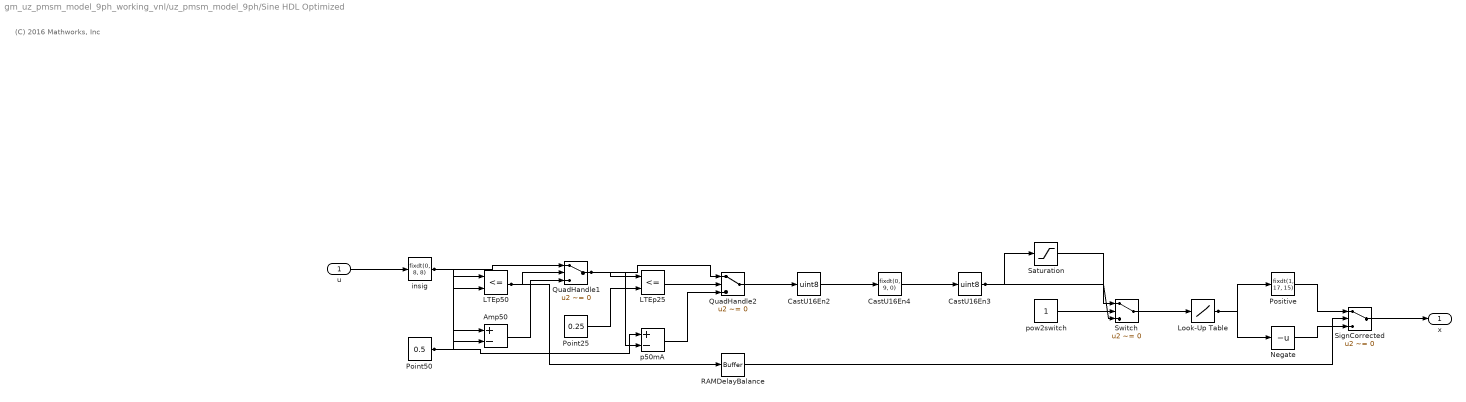
== system gm_uz_pmsm_model_9ph_working_vnl/uz_pmsm_model_9ph/Sine HDL Optimized ==
  note: (C) 2016 Mathworks, Inc
  u : Inport  OutDataTypeStr=fixdt(1, 25, 12)  SampleTime=2e-09
  Amp50 : Sum  Inputs=+-  AccumDataTypeStr=fixdt(1, 18, 17)  OutDataTypeStr=fixdt(1, 18, 17)  SampleTime=2e-09
  CastU16En2 : DataTypeConversion  OutDataTypeStr=uint8  ConvertRealWorld=Stored Integer (SI)  SampleTime=2e-09
  CastU16En3 : DataTypeConversion  OutDataTypeStr=uint8  ConvertRealWorld=Stored Integer (SI)  SampleTime=2e-09  SaturateOnIntegerOverflow=on
  CastU16En4 : DataTypeConversion  OutDataTypeStr=fixdt(0, 9, 0)  SampleTime=2e-09
  LTEp25 : RelationalOperator  Operator=<=  OutDataTypeStr=boolean  SampleTime=2e-09  RndMeth=Nearest
  LTEp50 : RelationalOperator  Operator=<=  OutDataTypeStr=boolean  SampleTime=2e-09  RndMeth=Nearest
  Look-Up Table : Lookup_n-D  NumberOfTableDimensions=1  BreakpointsForDimension1="fi(\"numerictype\",numerictype(0,8,0),\"fimath\",fimath(\"RoundingMethod\", \"Floor\",\"OverflowAction\", \"Wrap\",\"ProductMode\",\"FullPrecision\",\"SumMode\",\"FullPrecision\"),\"Value\",\"[0 1 2 3 4 5 6 7 8 9 10 11 12 13 14 15 16 17 18 19 20 21 22 23 24 25 26 27 28 29 30 31 32 33 34 35 36 37 38 39 40 41 42 43 44 45 46 47 48 49 50 51 52 53 54 55 56 57 58 59 60 61 62 63]\")"  Table="reshape(fi(\"numerictype\",numerictype(1,17,15),\"fimath\",fimath(\"RoundingMethod\", \"Floor\",\"OverflowAction\", \"Wrap\",\"ProductMode\",\"FullPrecision\",\"SumMode\",\"FullPrecision\"),\"Value\",\"[0;0.0245361328125;0.049072265625;0.073577880859375;0.0980224609375;0.122406005859375;0.146728515625;0.17095947265625;0.195098876953125;0.2191162109375;0.24298095703125;0.2667236328125;0.290283203125;0.313690185546875;0.336883544921875;0.359893798828125;0.3826904296875;0.405242919921875;0.42755126953125;0.449615478515625;0.471405029296875;0.492889404296875;0.51409912109375;0.535003662109375;0.555572509765625;0.5758056640625;0.595703125;0.615234375;0.6343994140625;0.653167724609375;0.67156982421875;0.689544677734375;0.70709228515625;0.7242431640625;0.740936279296875;0.7572021484375;0.77301025390625;0.788360595703125;0.80322265625;0.817596435546875;0.83148193359375;0.8448486328125;0.85772705078125;0.870086669921875;0.881927490234375;0.893218994140625;0.90399169921875;0.914215087890625;0.92388916015625;0.9329833984375;0.941558837890625;0.94952392578125;0.956939697265625;0.963775634765625;0.97003173828125;0.9757080078125;0.98077392578125;0.98529052734375;0.989166259765625;0.99249267578125;0.99517822265625;0.997283935546875;0.998809814453125;0.99969482421875]\"), [1  64])"  InterpMethod=Flat  ExtrapMethod=Clip  DiagnosticForOutOfRangeInput=Error  SampleTime=2e-09  OutDataTypeStr=fixdt(1, 17, 15)  InputSameDT=on
  Negate : UnaryMinus  SampleTime=2e-09
  Point25 : Constant  Value=0.25  OutDataTypeStr=fixdt(0, 17, 17)  SampleTime=2e-09
  Point50 : Constant  Value=0.5  OutDataTypeStr=fixdt(0, 17, 17)  SampleTime=2e-09
  Positive : DataTypeConversion  OutDataTypeStr=fixdt(1, 17, 15)  SampleTime=2e-09
  QuadHandle1 : Switch  Criteria=u2 ~= 0  Threshold=double(0)  OutDataTypeStr=fixdt(1, 18, 17)  SampleTime=2e-09
  QuadHandle2 : Switch  Criteria=u2 ~= 0  Threshold=double(0)  OutDataTypeStr=fixdt(0, 8, 8)  SampleTime=2e-09
  RAMDelayBalance : hdlmdlgenlib/Buffer
      settings: SourceProductBaseCode=SL
  Saturation : Saturate  UpperLimit="fi(0,0,8,0,\"hex\",\"3f\")"  LowerLimit="fi(0,0,8,0,\"hex\",\"00\")"  SampleTime=2e-09  OutDataTypeStr=uint8
  SignCorrected : Switch  Criteria=u2 ~= 0  Threshold=double(0)  OutDataTypeStr=fixdt(1, 17, 15)  SampleTime=2e-09
  Switch : Switch  Criteria=u2 ~= 0  Threshold=double(0)  OutDataTypeStr=uint8  SampleTime=2e-09
  insig : DataTypeConversion  OutDataTypeStr=fixdt(0, 8, 8)  SampleTime=2e-09
  p50mA : Sum  Inputs=+-  AccumDataTypeStr=fixdt(1, 19, 17)  OutDataTypeStr=fixdt(1, 19, 17)  SampleTime=2e-09
  pow2switch : Constant  OutDataTypeStr=boolean  SampleTime=2e-09
  x : Outport  SampleTime=2e-09
  wires:
  u/1 -> insig/1
  pow2switch/1 -> Switch/2
  p50mA/1 -> QuadHandle2/3
  insig/1 -> Amp50/1, LTEp50/1, QuadHandle1/1
  Switch/1 -> Look-Up Table/1
  SignCorrected/1 -> x/1
  Saturation/1 -> Switch/1
  RAMDelayBalance/1 -> SignCorrected/2
  QuadHandle2/1 -> CastU16En2/1
  QuadHandle1/1 -> LTEp25/1, QuadHandle2/1, p50mA/2
  Positive/1 -> SignCorrected/1
  Point50/1 -> Amp50/2, LTEp50/2, p50mA/1
  Point25/1 -> LTEp25/2
  Negate/1 -> SignCorrected/3
  Look-Up Table/1 -> Negate/1, Positive/1
  LTEp50/1 -> RAMDelayBalance/1, QuadHandle1/2
  LTEp25/1 -> QuadHandle2/2
  CastU16En4/1 -> CastU16En3/1
  CastU16En3/1 -> Saturation/1, Switch/3
  CastU16En2/1 -> CastU16En4/1
  Amp50/1 -> QuadHandle1/3

== system gm_uz_pmsm_model_9ph_working_vnl/uz_pmsm_model_9ph/Sum1 ==
  In1 : Inport
  In2 : Inport  Port=2
  Sum1 : Sum  Inputs=+-  OutDataTypeStr=single  SampleTime=2e-09
  Sum1_pd1 : Delay  DelayLength=6
  Out1 : Outport
  wires:
  Sum1_pd1/1 -> Out1/1
  Sum1/1 -> Sum1_pd1/1
  In2/1 -> Sum1/2
  In1/1 -> Sum1/1

== system gm_uz_pmsm_model_9ph_working_vnl/uz_pmsm_model_9ph/Sum1_stage2 ==
  In1 : Inport
  In2 : Inport  Port=2
  Sum1_stage2 : Sum  Inputs=+-  OutDataTypeStr=single  SampleTime=2e-09
  Sum1_stage2_pd1 : Delay  DelayLength=6
  Out1 : Outport
  wires:
  Sum1_stage2_pd1/1 -> Out1/1
  Sum1_stage2/1 -> Sum1_stage2_pd1/1
  In2/1 -> Sum1_stage2/2
  In1/1 -> Sum1_stage2/1

== system gm_uz_pmsm_model_9ph_working_vnl/uz_pmsm_model_9ph/Sum1_stage3 ==
  In1 : Inport
  In2 : Inport  Port=2
  Sum1_stage3 : Sum  Inputs=+-  OutDataTypeStr=single  SampleTime=2e-09
  Sum1_stage3_pd1 : Delay  DelayLength=6
  Out1 : Outport
  wires:
  Sum1_stage3_pd1/1 -> Out1/1
  Sum1_stage3/1 -> Sum1_stage3_pd1/1
  In2/1 -> Sum1_stage3/2
  In1/1 -> Sum1_stage3/1

== system gm_uz_pmsm_model_9ph_working_vnl/uz_pmsm_model_9ph/Sum2 ==
  In1 : Inport
  In2 : Inport  Port=2
  Sum2 : Sum  Inputs=+-  OutDataTypeStr=single  SampleTime=2e-09
  Sum2_pd1 : Delay  DelayLength=6
  Out1 : Outport
  wires:
  Sum2_pd1/1 -> Out1/1
  Sum2/1 -> Sum2_pd1/1
  In2/1 -> Sum2/2
  In1/1 -> Sum2/1

== system gm_uz_pmsm_model_9ph_working_vnl/uz_pmsm_model_9ph/Sum3 ==
  In1 : Inport
  In2 : Inport  Port=2
  Sum3 : Sum  OutDataTypeStr=double  SampleTime=2e-09
  Sum3_pd1 : Delay  DelayLength=6
  Out1 : Outport
  wires:
  Sum3_pd1/1 -> Out1/1
  Sum3/1 -> Sum3_pd1/1
  In2/1 -> Sum3/2
  In1/1 -> Sum3/1

== system gm_uz_pmsm_model_9ph_working_vnl/uz_pmsm_model_9ph/Sum31 ==
  In1 : Inport
  In2 : Inport  Port=2
  Sum31 : Sum  OutDataTypeStr=double  SampleTime=2e-09
  Sum31_pd1 : Delay  DelayLength=6
  Out1 : Outport
  wires:
  Sum31_pd1/1 -> Out1/1
  Sum31/1 -> Sum31_pd1/1
  In2/1 -> Sum31/2
  In1/1 -> Sum31/1

== system gm_uz_pmsm_model_9ph_working_vnl/uz_pmsm_model_9ph/Sum310 ==
  In1 : Inport
  In2 : Inport  Port=2
  Sum310 : Sum  OutDataTypeStr=double  SampleTime=2e-09
  Sum310_pd1 : Delay  DelayLength=6
  Out1 : Outport
  wires:
  Sum310_pd1/1 -> Out1/1
  Sum310/1 -> Sum310_pd1/1
  In2/1 -> Sum310/2
  In1/1 -> Sum310/1

== system gm_uz_pmsm_model_9ph_working_vnl/uz_pmsm_model_9ph/Sum32 ==
  In1 : Inport
  In2 : Inport  Port=2
  Sum32 : Sum  OutDataTypeStr=double  SampleTime=2e-09
  Sum32_pd1 : Delay  DelayLength=6
  Out1 : Outport
  wires:
  Sum32_pd1/1 -> Out1/1
  Sum32/1 -> Sum32_pd1/1
  In2/1 -> Sum32/2
  In1/1 -> Sum32/1

== system gm_uz_pmsm_model_9ph_working_vnl/uz_pmsm_model_9ph/Sum33 ==
  In1 : Inport
  In2 : Inport  Port=2
  Sum33 : Sum  Inputs=+-  OutDataTypeStr=single  SampleTime=2e-09
  Sum33_pd1 : Delay  DelayLength=6
  Out1 : Outport
  wires:
  Sum33_pd1/1 -> Out1/1
  Sum33/1 -> Sum33_pd1/1
  In2/1 -> Sum33/2
  In1/1 -> Sum33/1

== system gm_uz_pmsm_model_9ph_working_vnl/uz_pmsm_model_9ph/Sum34 ==
  In1 : Inport
  In2 : Inport  Port=2
  Sum34 : Sum  OutDataTypeStr=double  SampleTime=2e-09
  Sum34_pd1 : Delay  DelayLength=6
  Out1 : Outport
  wires:
  Sum34_pd1/1 -> Out1/1
  Sum34/1 -> Sum34_pd1/1
  In2/1 -> Sum34/2
  In1/1 -> Sum34/1

== system gm_uz_pmsm_model_9ph_working_vnl/uz_pmsm_model_9ph/Sum35 ==
  In1 : Inport
  In2 : Inport  Port=2
  Sum35 : Sum  OutDataTypeStr=double  SampleTime=2e-09
  Sum35_pd1 : Delay  DelayLength=6
  Out1 : Outport
  wires:
  Sum35_pd1/1 -> Out1/1
  Sum35/1 -> Sum35_pd1/1
  In2/1 -> Sum35/2
  In1/1 -> Sum35/1

== system gm_uz_pmsm_model_9ph_working_vnl/uz_pmsm_model_9ph/Sum36 ==
  In1 : Inport
  In2 : Inport  Port=2
  Sum36 : Sum  OutDataTypeStr=double  SampleTime=2e-09
  Sum36_pd1 : Delay  DelayLength=6
  Out1 : Outport
  wires:
  Sum36_pd1/1 -> Out1/1
  Sum36/1 -> Sum36_pd1/1
  In2/1 -> Sum36/2
  In1/1 -> Sum36/1

== system gm_uz_pmsm_model_9ph_working_vnl/uz_pmsm_model_9ph/Sum37 ==
  In1 : Inport
  In2 : Inport  Port=2
  Sum37 : Sum  OutDataTypeStr=double  SampleTime=2e-09
  Sum37_pd1 : Delay  DelayLength=6
  Out1 : Outport
  wires:
  Sum37_pd1/1 -> Out1/1
  Sum37/1 -> Sum37_pd1/1
  In2/1 -> Sum37/2
  In1/1 -> Sum37/1

== system gm_uz_pmsm_model_9ph_working_vnl/uz_pmsm_model_9ph/Sum38 ==
  In1 : Inport
  In2 : Inport  Port=2
  Sum38 : Sum  OutDataTypeStr=double  SampleTime=2e-09
  Sum38_pd1 : Delay  DelayLength=6
  Out1 : Outport
  wires:
  Sum38_pd1/1 -> Out1/1
  Sum38/1 -> Sum38_pd1/1
  In2/1 -> Sum38/2
  In1/1 -> Sum38/1

== system gm_uz_pmsm_model_9ph_working_vnl/uz_pmsm_model_9ph/Sum39 ==
  In1 : Inport
  In2 : Inport  Port=2
  Sum39 : Sum  OutDataTypeStr=double  SampleTime=2e-09
  Sum39_pd1 : Delay  DelayLength=6
  Out1 : Outport
  wires:
  Sum39_pd1/1 -> Out1/1
  Sum39/1 -> Sum39_pd1/1
  In2/1 -> Sum39/2
  In1/1 -> Sum39/1

== system gm_uz_pmsm_model_9ph_working_vnl/uz_pmsm_model_9ph/Sum_stage2 ==
  In1 : Inport
  In2 : Inport  Port=2
  Sum_stage2 : Sum  Inputs=+-  OutDataTypeStr=single  SampleTime=2e-09
  Sum_stage2_pd1 : Delay  DelayLength=6
  Out1 : Outport
  wires:
  Sum_stage2_pd1/1 -> Out1/1
  Sum_stage2/1 -> Sum_stage2_pd1/1
  In2/1 -> Sum_stage2/2
  In1/1 -> Sum_stage2/1

== system gm_uz_pmsm_model_9ph_working_vnl/uz_pmsm_model_9ph/Sum_stage3 ==
  In1 : Inport
  In2 : Inport  Port=2
  Sum_stage3 : Sum  OutDataTypeStr=single  SampleTime=2e-09
  Sum_stage3_pd1 : Delay  DelayLength=6
  Out1 : Outport
  wires:
  Sum_stage3_pd1/1 -> Out1/1
  Sum_stage3/1 -> Sum_stage3_pd1/1
  In2/1 -> Sum_stage3/2
  In1/1 -> Sum_stage3/1

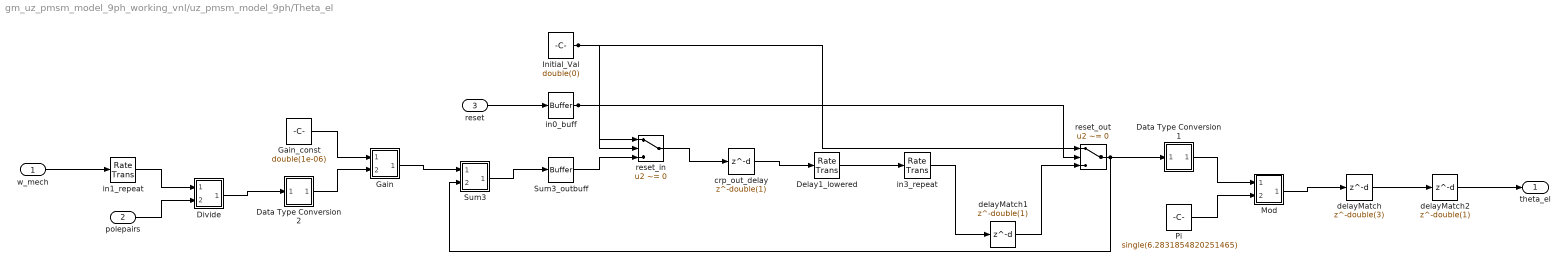
== system gm_uz_pmsm_model_9ph_working_vnl/uz_pmsm_model_9ph/Theta_el ==
  w_mech : Inport  OutDataTypeStr=single  PortDimensions=1  SampleTime=1e-06
  polepairs : Inport  Port=2  OutDataTypeStr=single  PortDimensions=1  SampleTime=2e-09
  reset : Inport  Port=3  OutDataTypeStr=boolean  PortDimensions=1  SampleTime=2e-09
  Data Type Conversion1 : Subsystem
      mask Display: disp('NFP\nconv');
  Data Type Conversion2 : Subsystem
      mask Display: disp('NFP\nconv');
  Delay1_lowered : RateTransition  OutPortSampleTimeOpt=Multiple of input port sample time  OutPortSampleTimeMultiple=500
  Divide : Subsystem
      mask Display: disp('NFP\nmul');
  Gain : Subsystem
      mask Display: disp('NFP\nmul');
  Gain_const : Constant  Value=double(1e-06)  OutDataTypeStr=double  SampleTime=2e-09
  Initial_Val : Constant  Value=double(0)  OutDataTypeStr=double  SampleTime=2e-09
  Mod : Subsystem
      mask Display: disp('NFP\nmath2');
  Pi : Constant  Value=single(6.2831854820251465)  OutDataTypeStr=single  SampleTime=2e-09
  Sum3 : Subsystem
      mask Display: disp('NFP\nadd');
  Sum3_outbuff : hdlmdlgenlib/Buffer
      settings: SourceProductBaseCode=SL
  crp_out_delay : Delay  DelayLength=double(1)  InitialCondition=0  SampleTime=2e-09
  delayMatch : Delay  DelayLength=double(3)  InitialCondition=0  SampleTime=2e-09
  delayMatch1 : Delay  DelayLength=double(1)  InitialCondition=0  SampleTime=2e-09
  delayMatch2 : Delay  DelayLength=double(1)  InitialCondition=0  SampleTime=2e-09
  in0_buff : hdlmdlgenlib/Buffer
      settings: SourceProductBaseCode=SL
  in1_repeat : RateTransition  Integrity=off  Deterministic=off  OutPortSampleTimeOpt=Multiple of input port sample time  OutPortSampleTimeMultiple=1/500
  in3_repeat : RateTransition  Integrity=off  Deterministic=off  OutPortSampleTimeOpt=Multiple of input port sample time  OutPortSampleTimeMultiple=1/500
  reset_in : Switch  Criteria=u2 ~= 0  Threshold=double(0)  OutDataTypeStr=double  SampleTime=2e-09
  reset_out : Switch  Criteria=u2 ~= 0  Threshold=double(0)  OutDataTypeStr=double  SampleTime=2e-09
  theta_el : Outport  SampleTime=2e-09
  wires:
  delayMatch/1 -> delayMatch2/1
  delayMatch1/1 -> reset_out/3
  in0_buff/1 -> reset_in/2, reset_out/2
  reset_out/1 -> Data Type Conversion1/1(In1), Sum3/2(In2)
  Gain/1(Out1) -> Sum3/1(In1)
  Data Type Conversion1/1(Out1) -> Mod/1(In1)
  Sum3/1(Out1) -> Sum3_outbuff/1
  Data Type Conversion2/1(Out1) -> Gain/2(In2)
  Divide/1(Out1) -> Data Type Conversion2/1(In1)
  Mod/1(Out1) -> delayMatch/1
  Gain_const/1 -> Gain/1(In1)
  reset_in/1 -> crp_out_delay/1
  Sum3_outbuff/1 -> reset_in/3
  Initial_Val/1 -> reset_in/1, reset_out/1
  Pi/1 -> Mod/2(In2)
  delayMatch2/1 -> theta_el/1
  in3_repeat/1 -> delayMatch1/1
  in1_repeat/1 -> Divide/1(In1)
  crp_out_delay/1 -> Delay1_lowered/1
  Delay1_lowered/1 -> in3_repeat/1
  reset/1 -> in0_buff/1
  polepairs/1 -> Divide/2(In2)
  w_mech/1 -> in1_repeat/1
